simulink model "bb_lqr_hg_sl"  (Simulink 8.7)
settings: Solver=FixedStepDiscrete  StartTime=0.0  StopTime=inf  FixedStep=ts  RelTol=1e-3
undefined symbols (not defined in the file): denlpf, F, numlpf, r1, ts
libraries: arduinolib x4, simulink x2
settings Model: Creator=hirata  LastModifiedBy=morita  SimulationMode=external  ExtModeTrigDuration=2
settings DataIOCC: SignalLoggingSaveFormat=ModelDataLogs
settings OptimizationCC: ExpressionDepthLimit=2147483647  OptimizeModelRefInitCode=on  LifeSpan=Inf  MaxStackSize=64
settings DebuggingCC: SolverPrmCheckMsg=warning  FcnCallInpInsideContextMsg=UseLocalSettings  StateNameClashWarn=warning
settings HardwareCC: ProdBitPerInt=16  ProdBitPerPointer=16  ProdIntDivRoundTo=Zero  ProdEndianess=LittleEndian  ProdWordSize=8  ProdHWDeviceType=Atmel->AVR  UseEmbeddedCoderFeatures=off  UseSimulinkCoderFeatures=off
settings RTWCC: SystemTargetFile=ert.tlc  HardwareBoard=Arduino Mega 2560  TLCOptions=-aInlineSetEventsForThisBaseRateFcn=TLC_FALSE -aSuppressMultiTaskScheduler=TLC_FALSE  TemplateMakefile=ert_default_tmf  Description=Embedded Coder  GenerateReport=on  Toolchain=Arduino AVR v1.6.1  BuildConfiguration=Faster Runs  IncludeHyperlinkInReport=on  LaunchReport=on  GenerateTraceInfo=on  GenerateTraceReport=on  GenerateTraceReportSl=on  GenerateTraceReportSf=on  GenerateTraceReportEml=on
settings MATStruct: className=codertarget.tools.BuildHook  argsTopModelOnly=[]  excludedModels=[]  includeReferencedModels=on  includeTopModel=on  enabled=on  UseCoderTarget=[1]  TargetHardware=Arduino Mega 2560  RTOS=Baremetal  Scheduler_interrupt_source=[0.0]  DataVersion=2016.02  Baudrate=115200  COMPort=codertarget.arduinobase.internal.getExternalModeMexArgs('Serial')  Verbose=[0]  IPAddress=codertarget.arduinobase.internal.getExternalModeMexArgs('Ethernet')  Port=17725  Configuration=Serial  BuildAction=Build, load and run  Set_host_COM_port=Automatically  COM_port_number=1  Enable_overrun_detection=[0.0]  Digital_output_to_set_on_overrun=13  Analog_input_reference_voltage=[0.0]  Serial0_baud_rate=9600  Serial1_baud_rate=9600  Serial2_baud_rate=9600  Serial3_baud_rate=9600  SPI_clock_out_frequency=4000  SPI_mode=Mode 0 - Clock Polarity 0, Clock Phase 0  SPI_bitorder=MSB first  Disable_DHCP_Ethernet=[0.0]  Local_ip_address=192.168.0.20  Local_mac_address=DE:AD:BE:EF:FE:ED  Disable_DHCP_Wifi=[0.0]  Wifi_ip_address=192.168.1.20  Wifi_SSID=yourNetwork  Set_Wifi_Encryption=None  Wifi_WEP_key=D0D0DEADF00DABBADEAFBEADED  Wifi_WEP_key_index=0  Wifi_WPA_password=secretPassword
settings CodeAppCC: ForceParamTrailComments=on  IgnoreCustomStorageClasses=off  OperatorAnnotations=on  SimulinkDataObjDesc=on  SFDataObjDesc=on  MATLABFcnDesc=on  InsertBlockDesc=on  MATLABSourceComments=on
settings ERTTargetCC: MultiwordLength=2048  SupportContinuousTime=on  SupportNonInlinedSFcns=on  SupportVariableSizeSignals=on

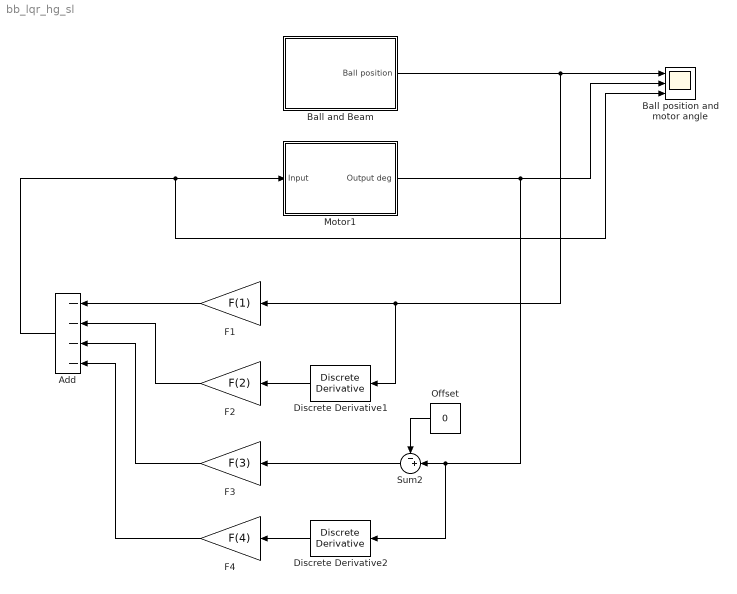
== system bb_lqr_hg_sl ==
  Add : Sum  Inputs=----
  Ball and Beam : Subsystem
  Ball position and motor angle : Scope  NumInputPorts=3
  Discrete Derivative1 : simulink/Discrete/Discrete Derivative  gainval=1.0  ICPrevScaledInput=0.0  InputProcessing=Inherited  OutMin=[]  OutMax=[]  OutDataType=fixdt(1, 16)  OutScaling=2^-10  DoSatur=off
  Discrete Derivative2 : simulink/Discrete/Discrete Derivative  gainval=1.0  ICPrevScaledInput=0.0  InputProcessing=Inherited  OutMin=[]  OutMax=[]  OutDataType=fixdt(1, 16)  OutScaling=2^-10  DoSatur=off
  F1 : Gain  Gain=F(1)
  F2 : Gain  Gain=F(2)
  F3 : Gain  Gain=F(3)
  F4 : Gain  Gain=F(4)
  Motor1 : Subsystem
  Offset : Constant  Value=0  SampleTime=ts
  Sum2 : Sum  Inputs=-+|
  wires:
  Discrete Derivative1/1 -> F2/1
  Discrete Derivative2/1 -> F4/1
  Ball and Beam/1(Ball position) -> Discrete Derivative1/1, F1/1, Ball position and motor angle/1
  Motor1/1(Output deg) -> Sum2/2, Discrete Derivative2/1, Ball position and motor angle/2
  F1/1 -> Add/1
  F2/1 -> Add/2
  F4/1 -> Add/4
  F3/1 -> Add/3
  Add/1 -> Motor1/1(Input), Ball position and motor angle/3
  Sum2/1 -> F3/1
  Offset/1 -> Sum2/1

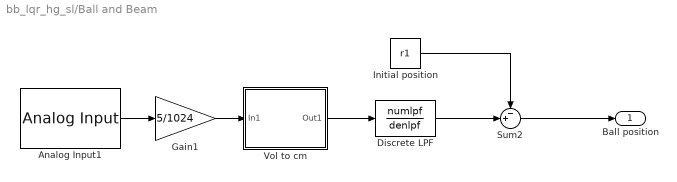
== system bb_lqr_hg_sl/Ball and Beam ==
  Analog Input1 : arduinolib/Analog Input  pinNumber=2  sampleTime=ts  blockPlatform=arduino
  Discrete LPF : DiscreteTransferFcn  Numerator=numlpf  Denominator=denlpf
  Gain1 : Gain  Gain=5/1024
  Initial position : Constant  Value=r1
  Sum2 : Sum  Inputs=-+|
  Vol to cm : Subsystem
  Ball position : Outport
  wires:
  Analog Input1/1 -> Gain1/1
  Gain1/1 -> Vol to cm/1(In1)
  Vol to cm/1(Out1) -> Discrete LPF/1
  Initial position/1 -> Sum2/1
  Discrete LPF/1 -> Sum2/2
  Sum2/1 -> Ball position/1

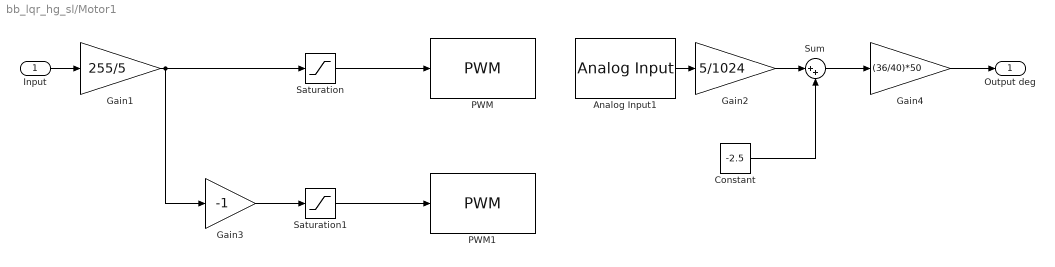
== system bb_lqr_hg_sl/Motor1 ==
  Input : Inport
  Analog Input1 : arduinolib/Analog Input  pinNumber=0  sampleTime=ts  blockPlatform=arduino
  Constant : Constant  Value=-2.5
  Gain1 : Gain  Gain=255/5
  Gain2 : Gain  Gain=5/1024
  Gain3 : Gain  Gain=-1
  Gain4 : Gain  Gain=(36/40)*50
  PWM : arduinolib/PWM  pinNumber=3  blockPlatform=arduino
  PWM1 : arduinolib/PWM  pinNumber=5  blockPlatform=arduino
  Saturation : Saturate  UpperLimit=255  LowerLimit=0
  Saturation1 : Saturate  UpperLimit=255  LowerLimit=0
  Sum : Sum  Inputs=|++
  Output deg : Outport
  wires:
  Input/1 -> Gain1/1
  Analog Input1/1 -> Gain2/1
  Saturation/1 -> PWM/1
  Gain1/1 -> Gain3/1, Saturation/1
  Saturation1/1 -> PWM1/1
  Gain4/1 -> Output deg/1
  Gain2/1 -> Sum/1
  Sum/1 -> Gain4/1
  Constant/1 -> Sum/2
  Gain3/1 -> Saturation1/1

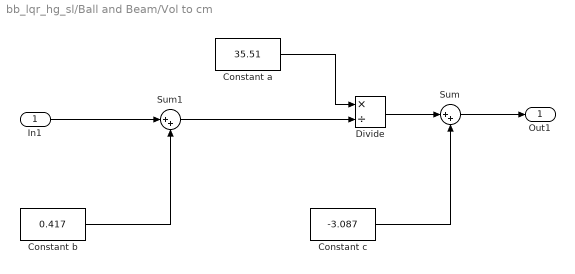
== system bb_lqr_hg_sl/Ball and Beam/Vol to cm ==
  In1 : Inport
  Constant a : Constant  Value=35.51
  Constant b : Constant  Value=0.417
  Constant c : Constant  Value=-3.087
  Divide : Product  Inputs=*/
  Sum : Sum  Inputs=|++
  Sum1 : Sum  Inputs=|++
  Out1 : Outport
  wires:
  Constant a/1 -> Divide/1
  Divide/1 -> Sum/1
  Sum/1 -> Out1/1
  Constant c/1 -> Sum/2
  In1/1 -> Sum1/1
  Sum1/1 -> Divide/2
  Constant b/1 -> Sum1/2
